simulink model "part6model"  (R2019b)
settings: Solver=VariableStepAuto  StartTime=0.0  StopTime=4  RelTol=1e-3
values from neighbouring files (symbols this model uses):
  A = [-2.6788 0;1 0]    [DC_Motor_Analysis.m]    (also in Part1.m = [[A11 A12];[A21 A22]]; SS_lab.m; mathModel.mat = [-2.28310502283  0; 1  0])
  B = [120.5465;0]    [DC_Motor_Analysis.m]    (also in Part1.m = [B1 B2].'; SS_lab.m = [12.05465;0]; mathModel.mat = [103.062962083 0])
  C = [0 1]    [DC_Motor_Analysis.m]    (also in Part1.m; mathModel.mat)
  encGain = (2*pi)/4096    (= 0.00153398078789)    [DC_Motor_Analysis.m]    (also in Part2.m; Part3.m; lqrPoles.mat; robust.mat)
  L_clo = place(A.', C.', [p p+.0001]).'    [Part5.m]    (also in Part6.m = place(A.', C.', p_des).')
settings Model: Creator=justinf  LastModifiedBy=justinf

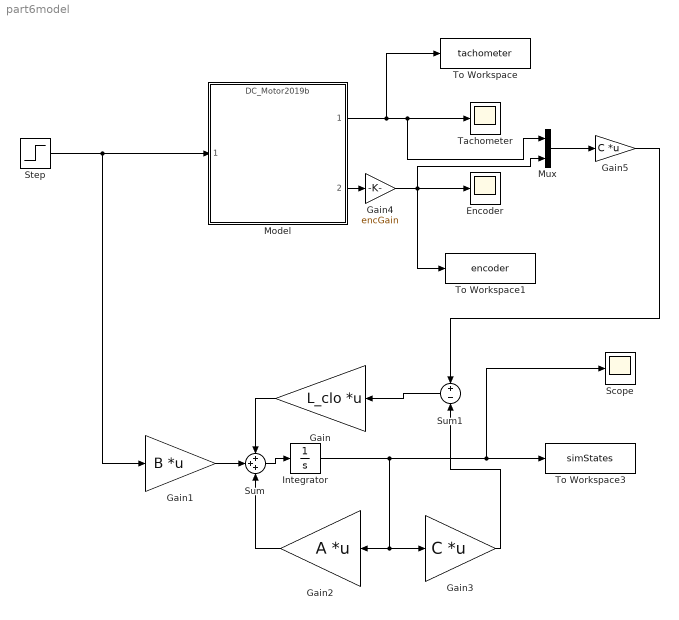
== system part6model ==
  Encoder : Scope
  Gain : Gain  Gain=L_clo  Multiplication=Matrix(K*u) (u vector)
  Gain1 : Gain  Gain=B  Multiplication=Matrix(K*u) (u vector)
  Gain2 : Gain  Gain=A  Multiplication=Matrix(K*u) (u vector)
  Gain3 : Gain  Gain=C  Multiplication=Matrix(K*u) (u vector)
  Gain4 : Gain  Gain=encGain
  Gain5 : Gain  Gain=C  Multiplication=Matrix(K*u) (u vector)
  Integrator : Integrator
  Model : ModelReference  ModelNameDialog=DC_Motor2019b.slxp  ModelReferenceVersion=1.20  CopyOfModelProtected=on
  Mux : Mux  Inputs=2
  Scope : Scope
  Step : Step  Time=0  After=.1  SampleTime=0
  Sum : Sum  Inputs=+++
  Sum1 : Sum  Inputs=+|-
  Tachometer : Scope
  To Workspace : ToWorkspace  VariableName=tachometer  SampleTime=-1
  To Workspace1 : ToWorkspace  VariableName=encoder  SampleTime=-1
  To Workspace3 : ToWorkspace  VariableName=simStates  SampleTime=-1
  wires:
  Model/1 -> To Workspace/1, Mux/1, Tachometer/1
  Step/1 -> Gain1/1, Model/1
  Gain1/1 -> Sum/2
  Gain2/1 -> Sum/3
  Gain/1 -> Sum/1
  Sum/1 -> Integrator/1
  Integrator/1 -> Gain2/1, Gain3/1, Scope/1, To Workspace3/1
  Sum1/1 -> Gain/1
  Gain3/1 -> Sum1/2
  Model/2 -> Gain4/1
  Gain4/1 -> Mux/2, To Workspace1/1, Encoder/1
  Mux/1 -> Gain5/1
  Gain5/1 -> Sum1/1
